simulink model "task_3_schem_2"  (R2024a)
settings: Solver=VariableStepAuto  StartTime=0.0  StopTime=10  RelTol=1e-3
undefined symbols (not defined in the file): A, B, B_s, C, D, F_H, G, G1, G2, G_s, init_g1, init_g2, invCM, K, Kn, M_H, T
settings Model: Creator=user  LastModifiedBy=user

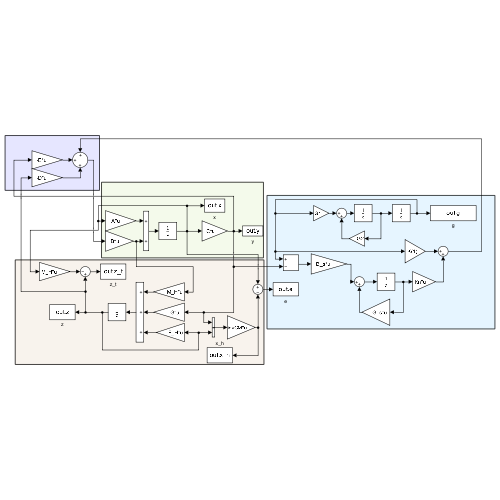
[thumbnail: Simulink's stored preview of the top-level diagram]
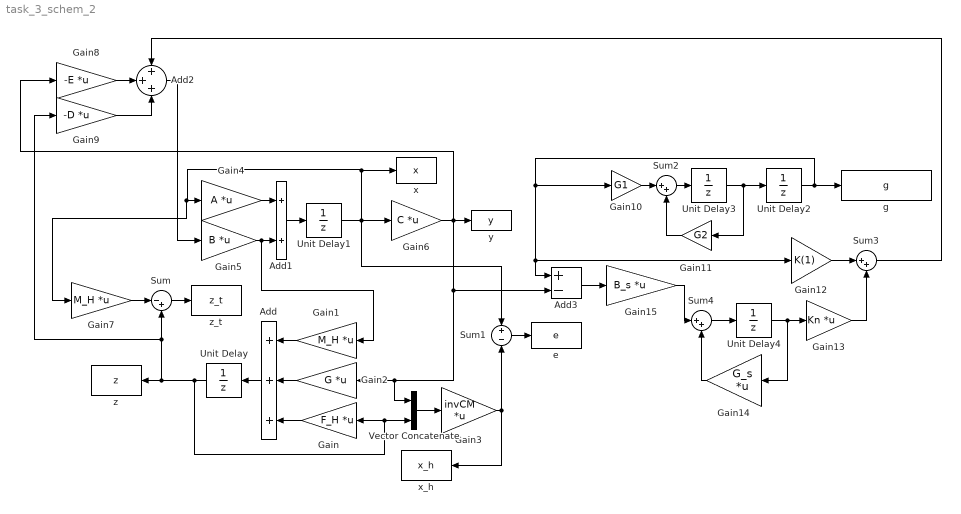
== system task_3_schem_2 ==
  Add : Sum  Inputs=+++
  Add1 : Sum
  Add2 : Sum  Inputs=+++
  Add3 : Sum  Inputs=+-
  Gain : Gain  Gain=F_H  Multiplication=Matrix(K*u)
  Gain1 : Gain  Gain=M_H  Multiplication=Matrix(K*u)
  Gain10 : Gain  Gain=G1
  Gain11 : Gain  Gain=G2
  Gain12 : Gain  Gain=K(1)
  Gain13 : Gain  Gain=Kn  Multiplication=Matrix(K*u)
  Gain14 : Gain  Gain=G_s  Multiplication=Matrix(K*u)
  Gain15 : Gain  Gain=B_s  Multiplication=Matrix(K*u)
  Gain2 : Gain  Gain=G  Multiplication=Matrix(K*u)
  Gain3 : Gain  Gain=invCM  Multiplication=Matrix(K*u)
  Gain4 : Gain  Gain=A  Multiplication=Matrix(K*u)
  Gain5 : Gain  Gain=B  Multiplication=Matrix(K*u)
  Gain6 : Gain  Gain=C  Multiplication=Matrix(K*u)
  Gain7 : Gain  Gain=M_H  Multiplication=Matrix(K*u)
  Gain8 : Gain  Gain=-E  Multiplication=Matrix(K*u)
  Gain9 : Gain  Gain=-D  Multiplication=Matrix(K*u)
  Sum : Sum  Inputs=|-+
  Sum1 : Sum  Inputs=+-
  Sum2 : Sum  Inputs=|++
  Sum3 : Sum  Inputs=|++
  Sum4 : Sum  Inputs=|++
  Unit Delay : UnitDelay  SampleTime=T  HasFrameUpgradeWarning=on
  Unit Delay1 : UnitDelay  InitialCondition=[1;1]  SampleTime=T  HasFrameUpgradeWarning=on
  Unit Delay2 : UnitDelay  InitialCondition=init_g2  SampleTime=T  HasFrameUpgradeWarning=on
  Unit Delay3 : UnitDelay  InitialCondition=init_g1  SampleTime=T  HasFrameUpgradeWarning=on
  Unit Delay4 : UnitDelay  SampleTime=T  HasFrameUpgradeWarning=on
  Vector Concatenate : Concatenate
  e : ToWorkspace  VariableName=e  SaveFormat=Timeseries  SampleTime=-1
  g : ToWorkspace  VariableName=g  SaveFormat=Timeseries  SampleTime=-1
  x : ToWorkspace  VariableName=x  SaveFormat=Timeseries  SampleTime=-1
  x_h : ToWorkspace  VariableName=x_h  SaveFormat=Timeseries  SampleTime=-1
  y : ToWorkspace  VariableName=y  SaveFormat=Timeseries  SampleTime=-1
  z : ToWorkspace  VariableName=z  SaveFormat=Timeseries  SampleTime=-1
  z_t : ToWorkspace  VariableName=z_t  SaveFormat=Timeseries  SampleTime=-1
  wires:
  Gain/1 -> Add/3
  Gain2/1 -> Add/2
  Gain1/1 -> Add/1
  Add/1 -> Unit Delay/1
  Unit Delay/1 -> Gain/1, Vector Concatenate/2, z/1, Gain9/1, Sum/2
  Vector Concatenate/1 -> Gain3/1
  Gain3/1 -> Sum1/2, x_h/1
  Gain4/1 -> Add1/1
  Gain5/1 -> Gain1/1, Add1/2
  Add1/1 -> Unit Delay1/1
  Unit Delay1/1 -> Sum1/1, Gain6/1, Gain7/1, Gain4/1, x/1
  Gain6/1 -> Gain8/1, y/1, Vector Concatenate/1, Gain2/1, Add3/2
  Gain7/1 -> Sum/1
  Sum1/1 -> e/1
  Gain9/1 -> Add2/3
  Add2/1 -> Gain5/1
  Gain8/1 -> Add2/2
  Gain11/1 -> Sum2/2
  Sum2/1 -> Unit Delay3/1
  Unit Delay3/1 -> Unit Delay2/1, Gain11/1
  Unit Delay2/1 -> Gain10/1, Gain12/1, Add3/1, g/1
  Gain10/1 -> Sum2/1
  Gain13/1 -> Sum3/2
  Gain15/1 -> Sum4/1
  Gain14/1 -> Sum4/2
  Sum4/1 -> Unit Delay4/1
  Unit Delay4/1 -> Gain14/1, Gain13/1
  Add3/1 -> Gain15/1
  Gain12/1 -> Sum3/1
  Sum3/1 -> Add2/1
  Sum/1 -> z_t/1
